simulink model "InnerOuter_Sim_newNav"  (Simulink 7.8)
settings: Solver=ode4  StartTime=0.0  StopTime=300  FixedStep=SampleT  RelTol=1e-3
InitFcn:
  | clc
  | innerOuterInit
values from neighbouring files (symbols this model uses):
  apSampleTime = 0.01    [innerOuterInit.m]
  SampleT = 0.005    [innerOuterInit.m]
  T = 0.01    [innerOuterInit.m]
undefined symbols (not defined in the file or in its folder): A1, Apolar, baseHeight, BasePoint, baseTemp, CD0, chord, CL0, CLa, CLa_dot, Clb, ClDa, CLDe, CLDf, ClDr, clock, Clp, CLq, Clr, Cm0, Cma, CmDe, CmDf, Cmq, Cnb, CnDa, CnDr, Cnp, Cnr, compensatorOn, CYb, CYDr, da_failamp, da_failbias, da_failper, daL_fail, daR_fail, deg, DiscIntNeverNeededParam, dr_fail, dr_failamp, dr_failbias, dr_failper, Earth, elarm, Euler_0, F, gaind, Init_onlyOnce, Init_Reset, ISA_g, Ixx, Iyy, Izz, L1OF, lapseRate, Light, mass, MIL, MinThK ... (+21)
libraries: simulink x69, aerolibconvert2 x19, SLUGS_Library x10, aerolibactuator x5, aerolibobsolete x3, dspmtrx3 x3, aerolibwind2 x2, aerolibtransform2 x1, aerolibatmos2 x1, dsPICdrivers x1
(part 2 of 3)

== system InnerOuter_Sim_newNav/BaroTest/Compute Barometric Height ==
  Base Height (m) : Inport
  Base Pressure (Pa) : Inport  Port=2
  Baro (Pa) : Inport  Port=3
  Constant2 : Constant  Value=baseTemp/(-LapseRate)  OutDataTypeStr=single
  Constant3 : Constant  Value=9.350253e-2  OutDataTypeStr=single
  Constant4 : Constant  Value=-1.888933e-1  OutDataTypeStr=single
  Constant5 : Constant  Value=2.180313e-5  OutDataTypeStr=single
  Divide : Product  Inputs=*/  OutDataTypeStr=single
  Divide{1..4} (4 alike) : Product  OutDataTypeStr=single
  Length Conversion : aerolibconvert2/Length Conversion  IU=ft  OU=m
  Sum1 : Sum  Inputs=|++  OutDataTypeStr=single
  Sum2 : Sum  Inputs=|+-  OutDataTypeStr=single
  Sum3 : Sum  Inputs=3  OutDataTypeStr=single
  "Altitude, m" : Outport
  wires:
  Length Conversion/1 -> Sum1/1
  Sum2/1 -> Divide/1
  Sum1/1 -> "Altitude, m"/1
  Divide3/1 -> Length Conversion/1
  Constant2/1 -> Divide3/2
  Sum3/1 -> Divide3/1
  Constant5/1 -> Sum3/3
  Divide2/1 -> Sum3/2
  Divide1/1 -> Sum3/1
  Constant4/1 -> Divide2/2
  Constant3/1 -> Divide1/2
  Divide4/1 -> Divide1/1  "x^2"
  Divide/1 -> Divide2/1, Divide4/1, Divide4/2  "x"
  Base Pressure (Pa)/1 -> Divide/2, Sum2/2
  Base Height (m)/1 -> Sum1/2
  Baro (Pa)/1 -> Sum2/1

== system InnerOuter_Sim_newNav/BaroTest/Initial Baro Bias ==
  Baro (Pa) : Inport
  Enable : EnablePort
  Data Type Conversion : DataTypeConversion  OutDataTypeStr=double
  Data Type Conversion1 : DataTypeConversion  OutDataTypeStr=single
  Low Pass8 : Subsystem  mask(DiscretizedZeroPole){Zeros=[], Poles=[-3], Gain=3, AbsTol=auto, SampleTime=.01, method=tustin, Wc=1}
      mask prompts: Zeros "Zeros (enter in s-main:)"; Poles "Poles (enter in s-domain:)"; Gain "Gain (enter in s-domain:)"; AbsTol "Absolute tolerance:"; SampleTime "Sample time:"; Wc "Critical Frequency (Hz):"
      mask help: Continuous mask uses c2d to transform parameters onto the Discrete Zero-Pole block inside.
      mask init:
      | st=SampleTime;
      | if length(st)>1
      |     st=SampleTime(1);
      | end
      | if(st>0)
      |     [zerosd,polesd,gaind] = sldiscutil('disczpk', {st,method,Wc,Zeros,Poles,Gain});
      | end	
      | s = get_param(gcb,'maskvalues');
      | zeross = s{1};
      | poless = s{2};
      | gainss = s{3};
      | %zerosc = eval(zeross);
      | %polesc = eval(poless);
      | %gainsc = eval(gainss);
      | sldiscutil('initzpkmask', st);
      | if(st==0)
      | set_param([gcb '/Zero Pole'], 'AbsoluteTolerance', AbsTol);
      | end
      mask StyleString: edit,edit,edit,edit,edit,popup(zoh|foh|tustin|prewarp|matched),edit
      mask CallbackString: |||||hidecrit|
      mask Display:
      | droots(zeross,poless,gainss)
      | text( 0.5, 1.0, method, 'verticalAlignment','top')
  Mux : Mux  Inputs=2
  Scope : Scope
      settings: SaveName=ScopeData8
  "[80k - 120k]" : Saturate  UpperLimit=120000  LowerLimit=80000
  Baro (Gnd) : Outport
  wires:
  Baro (Pa)/1 -> Data Type Conversion/1
  Low Pass8/1(Out1) -> Data Type Conversion1/1
  Data Type Conversion/1 -> Low Pass8/1(In1)
  Data Type Conversion1/1 -> Mux/2, "[80k - 120k]"/1
  Mux/1 -> Scope/1
  "[80k - 120k]"/1 -> Baro (Gnd)/1, Mux/1

== system InnerOuter_Sim_newNav/BaroTest/Zero Out Height ==
  Base Height : Inport
  Computed Height : Inport  Port=2
  Enable : EnablePort
  Integer Delay : Delay  DelayLength=1  InitialCondition=0  InputProcessing=Inherited  SampleTime=.01
  Sum : Sum  Inputs=|+-  OutDataTypeStr=single
  Height Offset : Outport
  wires:
  Computed Height/1 -> Integer Delay/1
  Sum/1 -> Height Offset/1
  Integer Delay/1 -> Sum/2
  Base Height/1 -> Sum/1

== system InnerOuter_Sim_newNav/Create ISR Location From WPs/get sim WP Coord from Index ==
  WP Idx : Inport
  Data Type Conversion : DataTypeConversion  OutDataTypeStr=double
  Data Type Conversion1 : DataTypeConversion  OutDataTypeStr=single
  MATLAB Fcn : MATLABFcn  MATLABFcn=Xpoints(u(1))  OutputDimensions=1  OutputSignalType=real
  MATLAB Fcn1 : MATLABFcn  MATLABFcn=Ypoints(u(1))  OutputDimensions=1
  MATLAB Fcn2 : MATLABFcn  MATLABFcn=Zpoints(u(1))  OutputDimensions=1
  Mux : Mux  Inputs=3
  WP Coord : Outport
  wires:
  Data Type Conversion/1 -> MATLAB Fcn2/1, MATLAB Fcn/1, MATLAB Fcn1/1
  MATLAB Fcn/1 -> Mux/1
  MATLAB Fcn1/1 -> Mux/2
  MATLAB Fcn2/1 -> Mux/3
  WP Idx/1 -> Data Type Conversion/1
  Mux/1 -> Data Type Conversion1/1
  Data Type Conversion1/1 -> WP Coord/1

== system InnerOuter_Sim_newNav/L1 Output Feedback Controller With  Projection Operator/Control  Law ==
  a : Inport
  u : Inport  Port=2
  Compute Coef : Subsystem
  Detect Change : Subsystem
  Divide : Product  SampleTime=apSampleTime
  Divide1 : Product  SampleTime=apSampleTime
  IC : InitialCondition
  Integer Delay : Delay  DelayLength=1  InputProcessing=Inherited  SampleTime=apSampleTime
  Integer Delay1 : Delay  DelayLength=1  InputProcessing=Inherited  SampleTime=apSampleTime
  Subtract : Sum  SampleTime=apSampleTime
  y : Outport
  wires:
  Integer Delay1/1 -> Divide1/2
  u/1 -> Integer Delay/1
  IC/1 -> Compute Coef/Enable
  Subtract/1 -> Integer Delay1/1, y/1
  Divide1/1 -> Subtract/2
  Divide/1 -> Subtract/1
  Integer Delay/1 -> Divide/2
  Detect Change/1(change?) -> IC/1
  Compute Coef/2(c) -> Divide1/1
  Compute Coef/1(b) -> Divide/1
  a/1 -> Detect Change/1(Data), Compute Coef/1(a)

== system InnerOuter_Sim_newNav/L1 Output Feedback Controller With  Projection Operator/Projection Operator ==
  Theta Max : Inport
  Eps 0 : Inport  Port=2
  Theta : Inport  Port=3
  y : Inport  Port=4
  Compare To Zero : simulink/Logic and Bit Operations/Compare To Zero  relop=>=  OutDataTypeStr=boolean  ZeroCross=off
  Compare To Zero1 : simulink/Logic and Bit Operations/Compare To Zero  relop=>  OutDataTypeStr=boolean  ZeroCross=off
  Data Type Conversion1 : DataTypeConversion
  Divide2 : Product  OutDataTypeStr=single
  Enabled Subsystem : Subsystem  TreatAsAtomicUnit=on
  Enabled Subsystem1 : Subsystem  TreatAsAtomicUnit=on
  Enabled Subsystem2 : Subsystem  TreatAsAtomicUnit=on
  F(theta) : Subsystem
  Logical Operator : Logic  Operator=NOT  AllPortsSameDT=off  OutDataTypeStr=uint(8)
  Logical Operator2 : Logic  AllPortsSameDT=off  OutDataTypeStr=uint(8)
  Merge : Merge  InitialOutput=0
  Scope1 : Scope  NumInputPorts=4
      settings: YMin=-0.6~-0.5~-100~-10  YMax=0~5~10~10  SaveName=ScopeData4
  Scope2 : Scope  NumInputPorts=2
      settings: TimeRange=400  YMin=-0.06~-0.06  YMax=0.06~0.06  SaveName=ScopeData15
  "y " : InportShadow  Port=4
  "y    " : InportShadow  Port=4
  "Proj(the, y)" : Outport
  wires:
  Enabled Subsystem1/1(Out1) -> Merge/2
  "y    "/1 -> Enabled Subsystem1/1(y), Enabled Subsystem2/1(y), Scope1/2
  Logical Operator/1 -> Enabled Subsystem/Enable, Scope2/2
  Logical Operator2/1 -> Logical Operator/1, Enabled Subsystem1/Enable, Enabled Subsystem2/Enable, Scope2/1
  Compare To Zero1/1 -> Logical Operator2/1
  F(theta)/2(dif_f_theta) -> Divide2/1, Enabled Subsystem1/3(grad), Enabled Subsystem2/3(grad), Scope1/4
  Compare To Zero/1 -> Logical Operator2/2
  Enabled Subsystem/1(Out1) -> Data Type Conversion1/1
  "y "/1 -> Enabled Subsystem/1(In1)
  Merge/1 -> "Proj(the, y)"/1
  Divide2/1 -> Compare To Zero1/1
  y/1 -> Divide2/2
  F(theta)/1(f_theta) -> Compare To Zero/1, Enabled Subsystem1/2(f_the), Enabled Subsystem2/2(f_the), Scope1/3
  Theta/1 -> F(theta)/3(Theta)
  Eps 0/1 -> F(theta)/2(Eps 0)
  Theta Max/1 -> F(theta)/1(Theta Max)
  Data Type Conversion1/1 -> Merge/1
  Enabled Subsystem2/1(Out1) -> Scope1/1

== system InnerOuter_Sim_newNav/L1 Output Feedback Controller With  Projection Operator/State Predictor ==
  a : Inport
  u : Inport  Port=2
  Compute Coef : Subsystem
  Detect Change : Subsystem
  Divide : Product  SampleTime=apSampleTime
  Divide1 : Product  SampleTime=apSampleTime
  IC : InitialCondition
  Integer Delay : Delay  DelayLength=1  InputProcessing=Inherited  SampleTime=apSampleTime
  Integer Delay1 : Delay  DelayLength=1  InputProcessing=Inherited  SampleTime=apSampleTime
  Subtract : Sum  SampleTime=apSampleTime
  y : Outport
  wires:
  a/1 -> Compute Coef/1(a), Detect Change/1(Data)
  Compute Coef/1(b) -> Divide/1
  Compute Coef/2(c) -> Divide1/1
  Detect Change/1(change?) -> IC/1
  Integer Delay/1 -> Divide/2
  Divide/1 -> Subtract/1
  Divide1/1 -> Subtract/2
  Subtract/1 -> y/1, Integer Delay1/1
  IC/1 -> Compute Coef/Enable
  u/1 -> Integer Delay/1
  Integer Delay1/1 -> Divide1/2

== system InnerOuter_Sim_newNav/L1 Output Feedback Controller With  Projection Operator/Trapezoidal Integrator ==
  x : Inport
  Reset : Inport  Port=2
  Constant : Constant  Value=1/3  OutDataTypeStr=single
  Constant1 : Constant  Value=4/3  OutDataTypeStr=single
  Constant2 : Constant  Value=T/2  OutDataTypeStr=single
  Constant3 : Constant  Value=1/3  OutDataTypeStr=single
  Constant5 : Constant  Value=0  OutDataTypeStr=single
  Integer Delay : Delay  DelayLength=1  InputProcessing=Inherited  SampleTime=T
  Integer Delay1 : Delay  InputProcessing=Inherited  SampleTime=T
  Integer Delay2 : Delay  DelayLength=1  InputProcessing=Inherited  SampleTime=T
  Product{,1..3} (4 alike) : Product  OutDataTypeStr=single  RndMeth=Zero
  Protect NaNs : Subsystem
  Protect NaNs1 : Subsystem
  Subtract : Sum  Inputs=3  OutDataTypeStr=single
  Subtract1 : Sum  Inputs=2  OutDataTypeStr=single
  Switch1 : Switch  Criteria=u2 > Threshold  Threshold=0.3  SampleTime=.01
  "[min max]" : Saturate  UpperLimit=upperLimit  LowerLimit=lowerLimit  SampleTime=T
  Int(x) : Outport
  wires:
  Protect NaNs1/1(Out1) -> Integer Delay2/1, Int(x)/1
  Protect NaNs/1(Out1) -> Integer Delay1/1, Integer Delay/1, Product/1
  Subtract1/1 -> "[min max]"/1
  Product3/1 -> Subtract1/2
  "[min max]"/1 -> Switch1/3
  Switch1/1 -> Protect NaNs1/1(In1)
  Reset/1 -> Switch1/2
  Constant5/1 -> Switch1/1
  Integer Delay2/1 -> Subtract1/1
  Subtract/1 -> Product3/2
  Constant2/1 -> Product3/1
  Product2/1 -> Subtract/3
  Product1/1 -> Subtract/2
  Product/1 -> Subtract/1
  x/1 -> Protect NaNs/1(In1)
  Constant3/1 -> Product2/2
  Integer Delay1/1 -> Product2/1
  Integer Delay/1 -> Product1/1
  Constant1/1 -> Product1/2
  Constant/1 -> Product/2

== system InnerOuter_Sim_newNav/PT Unit (Vlad) /LPF the Euler and Construct Matrix ==
  Euler : Inport
  Euler Angles to  Direction Cosine Matrix : aerolibobsolete/Euler Angles to  Direction Cosine Matrix
  Terminator : Terminator
  "Tustin Lowpass, Auto Initial Condition1" : Subsystem  mask(Tustin1stOrderLowpassAutoInitialCondition){f=75, T=T}
      mask prompts: f "Lowpass Frequency"; T "Sample Time"
      mask help: Takes a 3db rolloff frequency (in Hz, NOT radians/s) and a sample time. Performs a symbolic Tustin conversion and implements in a discrete filter. The initial output of the filter is set by the first sample.
      mask Help: Enter the desired 3db rolloff frequency in Hz and the sample time. Initial conditions are sampled automatically.
      mask Display: fprintf('%.2f Hz lowpass',f)
  "Tustin Lowpass, Auto Initial Condition2" : Subsystem  mask(Tustin1stOrderLowpassAutoInitialCondition){f=75, T=T}
      mask prompts: f "Lowpass Frequency"; T "Sample Time"
      mask help: Takes a 3db rolloff frequency (in Hz, NOT radians/s) and a sample time. Performs a symbolic Tustin conversion and implements in a discrete filter. The initial output of the filter is set by the first sample.
      mask Help: Enter the desired 3db rolloff frequency in Hz and the sample time. Initial conditions are sampled automatically.
      mask Display: fprintf('%.2f Hz lowpass',f)
  "Tustin Lowpass, Auto Initial Condition3" : Subsystem  mask(Tustin1stOrderLowpassAutoInitialCondition){f=75, T=T}
      mask prompts: f "Lowpass Frequency"; T "Sample Time"
      mask help: Takes a 3db rolloff frequency (in Hz, NOT radians/s) and a sample time. Performs a symbolic Tustin conversion and implements in a discrete filter. The initial output of the filter is set by the first sample.
      mask Help: Enter the desired 3db rolloff frequency in Hz and the sample time. Initial conditions are sampled automatically.
      mask Display: fprintf('%.2f Hz lowpass',f)
  "[a b c]" : Demux  Outputs=3
  myMux Fun5 : MATLAB Function  TreatAsAtomicUnit=on
  Rfg2b : Outport
  wires:
  myMux Fun5/1(y) -> Terminator/1
  Euler/1 -> Euler Angles to  Direction Cosine Matrix/1, "[a b c]"/1
  "[a b c]"/3 -> "Tustin Lowpass, Auto Initial Condition3"/1(In1)
  "[a b c]"/2 -> "Tustin Lowpass, Auto Initial Condition1"/1(In1)
  "[a b c]"/1 -> "Tustin Lowpass, Auto Initial Condition2"/1(In1)
  "Tustin Lowpass, Auto Initial Condition3"/1(Out1) -> myMux Fun5/3(u3)
  "Tustin Lowpass, Auto Initial Condition1"/1(Out1) -> myMux Fun5/2(u2)
  "Tustin Lowpass, Auto Initial Condition2"/1(Out1) -> myMux Fun5/1(u1)
  Euler Angles to  Direction Cosine Matrix/1 -> Rfg2b/1

== system InnerOuter_Sim_newNav/Simple Car Model/Heading/Speed to Velocity ==
  Heading : Inport
  Speed : Inport  Port=2
  Add : Sum  Inputs=+-
  Angle Conversion : aerolibconvert2/Angle Conversion  IU=deg  OU=rad
  Divide : Product
  Divide1 : Product
  Low pass the  change of direction : Subsystem  mask(Tustin1stOrderLowpassAutoInitialCondition){f=0.05, T=apSampleTime}
      mask prompts: f "Lowpass Frequency"; T "Sample Time"
      mask help: Takes a 3db rolloff frequency (in Hz, NOT radians/s) and a sample time. Performs a symbolic Tustin conversion and implements in a discrete filter. The initial output of the filter is set by the first sample.
      mask Help: Enter the desired 3db rolloff frequency in Hz and the sample time. Initial conditions are sampled automatically.
      mask Display: fprintf('%.2f Hz lowpass',f)
  Mux : Mux  Inputs=3
  Rate Transition1 : RateTransition  OutPortSampleTime=apSampleTime
  Rate Transition2 : RateTransition  OutPortSampleTime=apSampleTime
  Speed1 : Constant  Value=0
  Speed2 : Constant  Value=450*pi/180  SampleTime=0.01
  Trigonometric Function : Trigonometry  Operator=cos
  Trigonometric Function1 : Trigonometry
  Velocity : Outport
  wires:
  Speed1/1 -> Mux/3
  Speed2/1 -> Add/1
  Add/1 -> Trigonometric Function/1, Trigonometric Function1/1  "alpha"
  Trigonometric Function/1 -> Divide/1
  Speed/1 -> Rate Transition2/1
  Divide/1 -> Mux/1
  Angle Conversion/1 -> Add/2
  Divide1/1 -> Mux/2
  Trigonometric Function1/1 -> Divide1/2
  Low pass the  change of direction/1(Out1) -> Angle Conversion/1
  Heading/1 -> Rate Transition1/1
  Mux/1 -> Velocity/1
  Rate Transition1/1 -> Low pass the  change of direction/1(In1)
  Rate Transition2/1 -> Divide1/1, Divide/2

== system InnerOuter_Sim_newNav/Simple Car Model/Simple Car Model ==
  Velocity : Inport
  Constant13 : Constant  Value=BasePoint  OutDataTypeStr=single
  Data Type Conversion : DataTypeConversion  OutDataTypeStr=single
  Data Type Conversion1 : DataTypeConversion  OutDataTypeStr=single
  Discrete-Time Integrator : DiscreteIntegrator  InitialConditionSource=external  SampleTime=0.01  ICPrevOutput=DiscIntNeverNeededParam  ICPrevScaledInput=DiscIntNeverNeededParam
  p_cg : Outport
  wires:
  Velocity/1 -> Data Type Conversion1/1
  Constant13/1 -> Discrete-Time Integrator/2
  Discrete-Time Integrator/1 -> Data Type Conversion/1
  Data Type Conversion/1 -> p_cg/1
  Data Type Conversion1/1 -> Discrete-Time Integrator/1

== system InnerOuter_Sim_newNav/6DOF Model/Plant/6-DOF EOM ==
  "[F,M]" : Inport
  Vb Corr : Inport  Port=2
  Angular Rates : Integrator  InitialCondition=PQR_0'
  Demux1 : Demux  Outputs=2
  Euler Angles : Integrator  InitialCondition=Euler_0
  Get Euler Dot : Subsystem
      mask Display:
      | port_label('input', 1, 'p, q, r')
      | port_label('input', 2, 'Euler')
      | port_label('output', 1, 'Euler_dot')
  Mux : Mux  Inputs=[3;3]
  NED2NEU : Gain  Gain=[1 0 0;0 1 0;0 0 -1]  Multiplication=Matrix(K*u)  SaturateOnIntegerOverflow=on  OutDataTypeStr=Inherit: Same as input  ParamDataTypeStr=Inherit: Same as input
  Position : Integrator  InitialCondition=Pos_0'
  RB2L * Vb : Product  Multiplication=Matrix(*)  SaturateOnIntegerOverflow=on  InputSameDT=on  OutDataTypeStr=Inherit: Same as first input
  RB2LTP : Subsystem
  Velocities Body : Integrator  InitialCondition=Vb_0'
  "[V1,2,3,W1,2,3]" : Subsystem
  X,Y,Z (LTP) : Outport
  "Vx, Vy, Vz" : Outport  Port=2
  Euler : Outport  Port=3
  "p, q, r" : Outport  Port=4
  Vb : Outport  Port=5
  Ab meas : Outport  Port=6
  Euler_dot : Outport  Port=7
  wires:
  "[V1,2,3,W1,2,3]"/1("Acc_meas ") -> Ab meas/1
  Euler Angles/1 -> "[V1,2,3,W1,2,3]"/2(Euler), Get Euler Dot/2(Euler), Euler/1, RB2LTP/1(Euler)
  Demux1/1 -> Velocities Body/1
  "[V1,2,3,W1,2,3]"/2(V*dot) -> Demux1/1
  Demux1/2 -> Angular Rates/1
  "[F,M]"/1 -> "[V1,2,3,W1,2,3]"/1("[F ; M]")
  RB2LTP/1(Rot) -> RB2L * Vb/1
  Velocities Body/1 -> Vb/1, RB2L * Vb/2
  Mux/1 -> "[V1,2,3,W1,2,3]"/3(V*)
  Position/1 -> X,Y,Z (LTP)/1
  Angular Rates/1 -> Get Euler Dot/1(p,q,r), Mux/2, "p, q, r"/1
  RB2L * Vb/1 -> NED2NEU/1, "Vx, Vy, Vz"/1  "NED"
  NED2NEU/1 -> Position/1
  Get Euler Dot/1(Euler_dot) -> Euler Angles/1, Euler_dot/1
  Vb Corr/1 -> Mux/1

== system InnerOuter_Sim_newNav/6DOF Model/Plant/Engine Model ==
  dt : Inport
  Vmag : Inport  Port=2
  Constant4 : Constant  Value=0
  Get To1 : Subsystem
  Mux : Mux  Inputs=2
  Mux1 : Mux  Inputs=3
  Thrust Available (lbs) : Fcn  Expr=u(1) - 0.047*sqrt(u(1))*u(2)
  kg2N : Gain  Gain=ISA_g  SaturateOnIntegerOverflow=on  OutDataTypeStr=Inherit: Same as input  ParamDataTypeStr=Inherit: Same as input
  lbs2kg : Gain  Gain=0.45359237  SaturateOnIntegerOverflow=on  OutDataTypeStr=Inherit: Same as input  ParamDataTypeStr=Inherit: Same as input
  Thrust : Outport
  wires:
  dt/1 -> Get To1/1(dt)
  Get To1/1(To) -> Mux/1
  Mux/1 -> Thrust Available (lbs)/1
  Thrust Available (lbs)/1 -> lbs2kg/1
  Vmag/1 -> Mux/2
  Mux1/1 -> Thrust/1
  lbs2kg/1 -> kg2N/1
  Constant4/1 -> Mux1/2, Mux1/3
  kg2N/1 -> Mux1/1

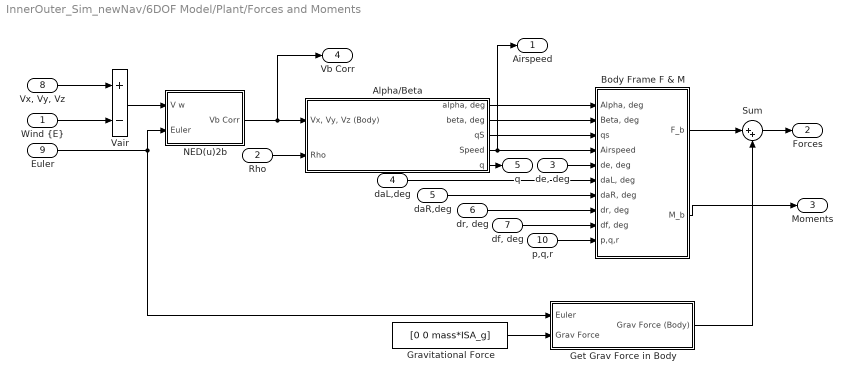
== system InnerOuter_Sim_newNav/6DOF Model/Plant/Forces and Moments ==
  "Wind {E}" : Inport
  Rho : Inport  Port=2
  "de, deg" : Inport  Port=3
  daL,deg : Inport  Port=4
  daR,deg : Inport  Port=5
  "dr, deg" : Inport  Port=6
  "df, deg" : Inport  Port=7
  "Vx, Vy, Vz " : Inport  Port=8
  Euler : Inport  Port=9  PortDimensions=3
  p,q,r : Inport  Port=10
  Alpha/Beta : Subsystem
  Body Frame F & M : Subsystem
  Get Grav Force in Body : Subsystem
  Gravitational Force : Constant  Value=[0 0 mass*ISA_g]  VectorParams1D=off
  NED(u)2b : Subsystem
  Sum : Sum  Inputs=|++  SaturateOnIntegerOverflow=on
  Vair : Sum  Inputs=+-  SaturateOnIntegerOverflow=on  InputSameDT=on  OutDataTypeStr=Inherit: Same as first input
  Airspeed : Outport
  Forces : Outport  Port=2
  Moments : Outport  Port=3
  Vb Corr : Outport  Port=4
  q : Outport  Port=5
  wires:
  Get Grav Force in Body/1(Grav Force (Body)) -> Sum/2
  Alpha/Beta/5(q) -> q/1
  "Vx, Vy, Vz "/1 -> Vair/1
  Vair/1 -> NED(u)2b/1(V w)
  Euler/1 -> NED(u)2b/2(Euler), Get Grav Force in Body/1(Euler)
  Rho/1 -> Alpha/Beta/2(Rho)
  NED(u)2b/1(Vb Corr) -> Alpha/Beta/1("Vx, Vy, Vz (Body)"), Vb Corr/1
  Body Frame F & M/2(M_b) -> Moments/1
  Gravitational Force/1 -> Get Grav Force in Body/2(Grav Force)
  Body Frame F & M/1(F_b) -> Sum/1
  Sum/1 -> Forces/1
  Alpha/Beta/3(qS) -> Body Frame F & M/3(qs)
  Alpha/Beta/4(Speed) -> Body Frame F & M/4(Airspeed), Airspeed/1
  "df, deg"/1 -> Body Frame F & M/9("df, deg")
  p,q,r/1 -> Body Frame F & M/10(p,q,r)
  Alpha/Beta/2("beta, deg") -> Body Frame F & M/2("Beta, deg")
  "dr, deg"/1 -> Body Frame F & M/8("dr, deg")
  daL,deg/1 -> Body Frame F & M/6("daL, deg")
  Alpha/Beta/1("alpha, deg") -> Body Frame F & M/1("Alpha, deg")
  "de, deg"/1 -> Body Frame F & M/5("de, deg")
  "Wind {E}"/1 -> Vair/2
  daR,deg/1 -> Body Frame F & M/7("daR, deg")

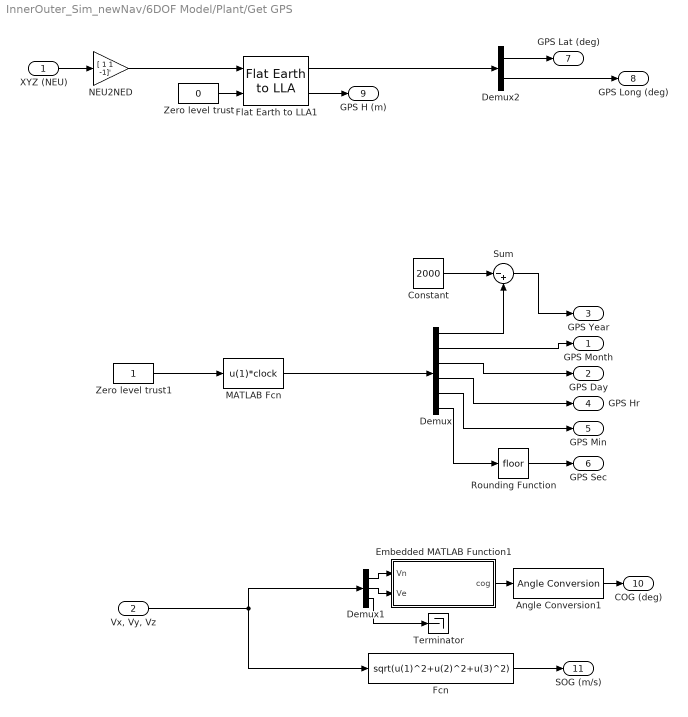
== system InnerOuter_Sim_newNav/6DOF Model/Plant/Get GPS ==
  XYZ (NEU) : Inport
  "Vx, Vy, Vz" : Inport  Port=2
  Angle Conversion1 : aerolibconvert2/Angle Conversion  IU=rad  OU=deg
  Constant : Constant  Value=2000
  Demux : Demux  Outputs=6
  Demux1 : Demux  Outputs=3
  Demux2 : Demux  Outputs=2
  Embedded MATLAB Function1 : MATLAB Function  TreatAsAtomicUnit=on
  Fcn : Fcn  Expr=sqrt(u(1)^2+u(2)^2+u(3)^2)
  Flat Earth to LLA1 : aerolibtransform2/Flat Earth to LLA  units=Metric (MKS)  ptype=Earth (WGS84)  F=1/298.257223563  R=6378137  LL0=[0 10]  psi=0
  MATLAB Fcn : MATLABFcn  MATLABFcn=u(1)*clock  OutputSignalType=real  SampleTime=SampleT
  NEU2NED : Gain  Gain=[ 1 1 -1]'  SaturateOnIntegerOverflow=on  OutDataTypeStr=Inherit: Same as input  ParamDataTypeStr=Inherit: Same as input
  Rounding Function : Rounding
  Sum : Sum  Inputs=|-+
  Terminator : Terminator
  Zero level trust : Constant  Value=0  SampleTime=SampleT
  Zero level trust1 : Constant  SampleTime=SampleT
  GPS Month : Outport
  GPS Day : Outport  Port=2
  GPS Year : Outport  Port=3
  GPS Hr : Outport  Port=4
  GPS Min : Outport  Port=5
  GPS Sec : Outport  Port=6
  GPS Lat (deg) : Outport  Port=7
  GPS Long (deg) : Outport  Port=8
  GPS H (m) : Outport  Port=9
  COG (deg) : Outport  Port=10
  SOG (m/s) : Outport  Port=11
  wires:
  NEU2NED/1 -> Flat Earth to LLA1/1
  Zero level trust/1 -> Flat Earth to LLA1/2
  XYZ (NEU)/1 -> NEU2NED/1
  Flat Earth to LLA1/1 -> Demux2/1
  Flat Earth to LLA1/2 -> GPS H (m)/1
  Zero level trust1/1 -> MATLAB Fcn/1
  MATLAB Fcn/1 -> Demux/1
  Demux/2 -> GPS Month/1
  Demux/3 -> GPS Day/1
  Demux/4 -> GPS Hr/1
  Demux/5 -> GPS Min/1
  Demux/6 -> Rounding Function/1
  Rounding Function/1 -> GPS Sec/1
  Demux2/1 -> GPS Lat (deg)/1
  Demux2/2 -> GPS Long (deg)/1
  Fcn/1 -> SOG (m/s)/1
  Demux1/1 -> Embedded MATLAB Function1/1(Vn)
  Demux1/2 -> Embedded MATLAB Function1/2(Ve)
  "Vx, Vy, Vz"/1 -> Demux1/1, Fcn/1
  Embedded MATLAB Function1/1(cog) -> Angle Conversion1/1
  Angle Conversion1/1 -> COG (deg)/1
  Demux/1 -> Sum/2
  Constant/1 -> Sum/1
  Sum/1 -> GPS Year/1
  Demux1/3 -> Terminator/1

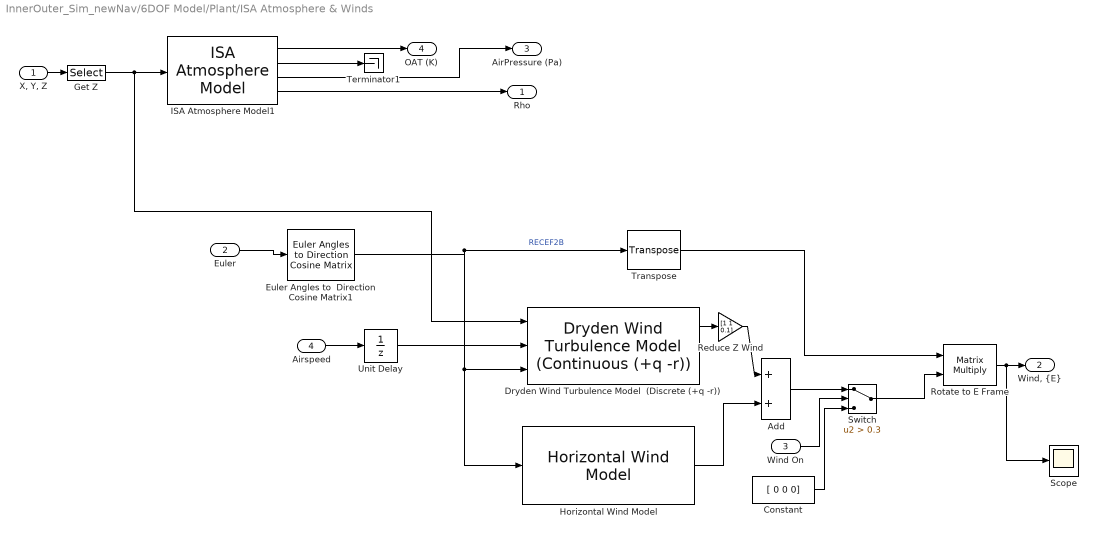
== system InnerOuter_Sim_newNav/6DOF Model/Plant/ISA Atmosphere & Winds ==
  "X, Y, Z" : Inport
  Euler : Inport  Port=2
  Wind On : Inport  Port=3
  Airspeed : Inport  Port=4
  Add : Sum  Inputs=2
  Constant : Constant  Value=[ 0 0 0]
  Dryden Wind Turbulence Model  (Discrete (+q -r)) : aerolibwind2/Dryden Wind Turbulence Model  (Continuous (+q -r))  units=Metric (MKS)  spec=MIL-F-8785C  model=Discrete Dryden (+q -r)  W20=windBase*0.3  Wdeg=windDirTurb  TurbProb=10^-2 - Light  L_high=533.4  Wingspan=span  ts=0.005  Seed=[23341 23342 23343 23344]  T_on=on
  Euler Angles to  Direction Cosine Matrix1 : aerolibobsolete/Euler Angles to  Direction Cosine Matrix
  Get Z : Selector  InputPortWidth=3  IndexOptions=Index vector (dialog)  Indices=[3]  OutputSizes=[(-2)]
  Horizontal Wind Model : aerolibwind2/Horizontal Wind Model  units=Metric (MKS)  Vw_source=Internal  Vwind=windBase  W_source=Internal  Wdeg=windDirHor
  ISA Atmosphere Model1 : aerolibatmos2/ISA Atmosphere Model  custom=off  g=9.80665  gamma=1.4  R=287.0531  L=0.0065  h_trop=11000  h_strat=20000  rho0=1.225  P0=101325  T0=288.15
  Reduce Z Wind : Gain  Gain=[1 1 0.1]
  Rotate to E Frame : Product  Multiplication=Matrix(*)
  Scope : Scope
      settings: YMin=-1  YMax=13  SaveName=windData  DataFormat=Array
  Switch : Switch  Criteria=u2 > Threshold  Threshold=0.3
  Terminator1 : Terminator
  Transpose : dspmtrx3/Transpose  Hermitian=off  overflowFlag=off
  Unit Delay : UnitDelay  SampleTime=-1
  Rho : Outport
  "Wind, {E}" : Outport  Port=2
  AirPressure (Pa) : Outport  Port=3
  OAT (K) : Outport  Port=4
  wires:
  "X, Y, Z"/1 -> Get Z/1
  Get Z/1 -> ISA Atmosphere Model1/1, Dryden Wind Turbulence Model  (Discrete (+q -r))/1
  ISA Atmosphere Model1/4 -> Rho/1
  ISA Atmosphere Model1/1 -> OAT (K)/1
  ISA Atmosphere Model1/2 -> Terminator1/1
  ISA Atmosphere Model1/3 -> AirPressure (Pa)/1
  Euler/1 -> Euler Angles to  Direction Cosine Matrix1/1
  Euler Angles to  Direction Cosine Matrix1/1 -> Dryden Wind Turbulence Model  (Discrete (+q -r))/3, Horizontal Wind Model/1, Transpose/1  "RECEF2B"
  Airspeed/1 -> Unit Delay/1
  Add/1 -> Switch/1
  Unit Delay/1 -> Dryden Wind Turbulence Model  (Discrete (+q -r))/2
  Horizontal Wind Model/1 -> Add/2
  Switch/1 -> Rotate to E Frame/2
  Wind On/1 -> Switch/2
  Constant/1 -> Switch/3
  Transpose/1 -> Rotate to E Frame/1
  Rotate to E Frame/1 -> "Wind, {E}"/1, Scope/1
  Dryden Wind Turbulence Model  (Discrete (+q -r))/1 -> Reduce Z Wind/1
  Reduce Z Wind/1 -> Add/1

== system InnerOuter_Sim_newNav/6DOF Model/Plant/Magnetometer ==
  Euler : Inport
  LTP2B : dspmtrx3/Transpose  Hermitian=off  overflowFlag=off
  Mag Field in nT source:  http://www.ngdc.noaa.gov/geomagmodels/struts/calcIGRFWMM : Constant  Value=magField
  Product : Product  Multiplication=Matrix(*)  RndMeth=Zero
  RB2LTP : Subsystem
  "Mag, nT" : Outport
  wires:
  RB2LTP/1(Rot) -> LTP2B/1
  LTP2B/1 -> Product/1
  Mag Field in nT source:  http://www.ngdc.noaa.gov/geomagmodels/struts/calcIGRFWMM/1 -> Product/2
  Euler/1 -> RB2LTP/1(Euler)
  Product/1 -> "Mag, nT"/1

== system InnerOuter_Sim_newNav/6DOF Model/Plant/[0, pi] Wrap Around ==
  Euler : Inport
  Compare To Zero : simulink/Logic and Bit Operations/Compare To Zero  relop=>=  OutDataTypeStr=uint8  ZeroCross=off
  Logical Operator : Logic  Operator=NOT  AllPortsSameDT=off  OutDataTypeStr=boolean
  Merge : Merge
  Mux2 : Mux  Inputs=2
  Negative Yaw : Subsystem
  Positive Yaw : Subsystem
  Selector1 : Selector  InputPortWidth=3  IndexOptions=Index vector (dialog)  Indices=[1 2]  OutputSizes=1
  Selector2 : Selector  InputPortWidth=3  IndexOptions=Index vector (dialog)  Indices=[3]  OutputSizes=1
  Euler-Wrapped : Outport
  wires:
  Euler/1 -> Selector2/1, Selector1/1
  Selector1/1 -> Mux2/1
  Mux2/1 -> Euler-Wrapped/1
  Selector2/1 -> Compare To Zero/1, Positive Yaw/1(yaw), Negative Yaw/1(yaw)
  Compare To Zero/1 -> Positive Yaw/Enable, Logical Operator/1
  Logical Operator/1 -> Negative Yaw/Enable
  Merge/1 -> Mux2/2
  Positive Yaw/1(yaw_wr) -> Merge/1
  Negative Yaw/1(yaw_wr) -> Merge/2

== system InnerOuter_Sim_newNav/6DOF Model/Split Ailerons And Introduce Failures/Aileron Flaping Failure ==
  Pulse Generator1 : DiscretePulseGenerator  PulseType=Time based  Amplitude=da_failamp  Period=da_failper  PulseWidth=50
  Vair2 : Sum  Inputs=+++  SaturateOnIntegerOverflow=on  InputSameDT=on  OutDataTypeStr=Inherit: Same as first input
  da_failbias : Constant  Value=da_failbias
  da_failbias1 : Constant  Value=0
  "da, Fail, deg" : Outport
  wires:
  Pulse Generator1/1 -> Vair2/1
  da_failbias/1 -> Vair2/2
  da_failbias1/1 -> Vair2/3
  Vair2/1 -> "da, Fail, deg"/1

== system InnerOuter_Sim_newNav/6DOF Model/Split Ailerons And Introduce Failures/Rudder Failure ==
  Pulse Generator1 : DiscretePulseGenerator  PulseType=Time based  Amplitude=dr_failamp  Period=dr_failper  PulseWidth=50
  Vair2 : Sum  Inputs=+++  SaturateOnIntegerOverflow=on  InputSameDT=on  OutDataTypeStr=Inherit: Same as first input
  da_failbias : Constant  Value=dr_failbias
  da_failbias1 : Constant  Value=0
  "da, Fail, deg" : Outport
  wires:
  Vair2/1 -> "da, Fail, deg"/1
  da_failbias1/1 -> Vair2/3
  da_failbias/1 -> Vair2/2
  Pulse Generator1/1 -> Vair2/1

== system InnerOuter_Sim_newNav/BaroTest/Initial Baro Bias/Low Pass8 ==
  In1 : Inport
  Discrete Zero-Pole : DiscreteZeroPole  Zeros=zerosd  Poles=polesd  Gain=gaind  SampleTime=SampleTime
  Out1 : Outport
  wires:
  In1/1 -> Discrete Zero-Pole/1
  Discrete Zero-Pole/1 -> Out1/1

== system InnerOuter_Sim_newNav/L1 Output Feedback Controller With  Projection Operator/Control  Law/Compute Coef ==
  a : Inport
  Enable : EnablePort
  -T : Gain  Gain=-apSampleTime  SampleTime=apSampleTime
  1-c : Sum  Inputs=-+  OutDataTypeStr=single  SampleTime=apSampleTime
  Constant : Constant
  Subsystem11 : Subsystem  AncestorBlock=SLUGS_Library/Subsystem11
  b : Outport
  c : Outport  Port=2
  wires:
  a/1 -> -T/1
  1-c/1 -> b/1
  Constant/1 -> 1-c/2
  Subsystem11/1(exp(u)) -> c/1, 1-c/1  "c"
  -T/1 -> Subsystem11/1(u)

== system InnerOuter_Sim_newNav/L1 Output Feedback Controller With  Projection Operator/Control  Law/Detect Change ==
  Data : Inport
  Abs1 : Abs  SampleTime=apSampleTime
  Difference1 : simulink/Discrete/Difference  ICPrevInput=0.0  InputProcessing=Inherited  OutMin=[]  OutMax=[]  OutDataType=sfix(16)  OutScaling=2^-10  DoSatur=off
  Saturation1 : Saturate  UpperLimit=1  LowerLimit=0  SampleTime=apSampleTime
  change? : Outport
  wires:
  Saturation1/1 -> change?/1
  Data/1 -> Difference1/1
  Abs1/1 -> Saturation1/1
  Difference1/1 -> Abs1/1

== system InnerOuter_Sim_newNav/L1 Output Feedback Controller With  Projection Operator/Projection Operator/Enabled Subsystem ==
  In1 : Inport
  Enable : EnablePort
  Out1 : Outport
  wires:
  In1/1 -> Out1/1

== system InnerOuter_Sim_newNav/L1 Output Feedback Controller With  Projection Operator/Projection Operator/Enabled Subsystem1 ==
  y : Inport
  f_the : Inport  Port=2
  grad : Inport  Port=3
  Enable : EnablePort
  Constant : Constant  OutDataTypeStr=single
  Divide1 : Product  OutDataTypeStr=single
  Divide2 : Product  OutDataTypeStr=single
  Sign : Signum
  Subtract : Sum  Inputs=+-  OutDataTypeStr=single
  Out1 : Outport
  wires:
  Divide2/1 -> Out1/1
  y/1 -> Divide2/1
  Subtract/1 -> Divide2/2
  f_the/1 -> Divide1/1
  Constant/1 -> Subtract/1
  Sign/1 -> Divide1/2
  grad/1 -> Sign/1
  Divide1/1 -> Subtract/2

== system InnerOuter_Sim_newNav/L1 Output Feedback Controller With  Projection Operator/Projection Operator/Enabled Subsystem2 ==
  y : Inport
  f_the : Inport  Port=2
  grad : Inport  Port=3
  Enable : EnablePort
  Constant : Constant  OutDataTypeStr=single
  Divide1 : Product  OutDataTypeStr=single
  Divide2 : Product  OutDataTypeStr=single
  Sign : Signum
  Subtract : Sum  Inputs=+-  OutDataTypeStr=single
  Out1 : Outport
  wires:
  Divide1/1 -> Subtract/2
  grad/1 -> Sign/1
  Sign/1 -> Divide1/2
  Constant/1 -> Subtract/1
  f_the/1 -> Divide1/1
  Subtract/1 -> Divide2/2
  y/1 -> Divide2/1
  Divide2/1 -> Out1/1

== system InnerOuter_Sim_newNav/L1 Output Feedback Controller With  Projection Operator/Projection Operator/F(theta) ==
  Theta Max : Inport
  Eps 0 : Inport  Port=2
  Theta : Inport  Port=3
  Constant : Constant  Value=2  OutDataTypeStr=single
  Divide : Product  OutDataTypeStr=single
  Divide1 : Product  OutDataTypeStr=single
  Divide2 : Product  OutDataTypeStr=single
  Divide3 : Product  Inputs=*/  OutDataTypeStr=single
  Divide4 : Product  Inputs=/**  OutDataTypeStr=single
  Subtract : Sum  Inputs=+-  OutDataTypeStr=single
  "Theta " : InportShadow  Port=3
  f_theta : Outport
  dif_f_theta : Outport  Port=2
  wires:
  Divide4/1 -> dif_f_theta/1
  "Theta "/1 -> Divide4/2
  Constant/1 -> Divide4/3
  Divide3/1 -> f_theta/1
  Divide2/1 -> Divide4/1, Divide3/2
  Subtract/1 -> Divide3/1
  Eps 0/1 -> Divide2/2
  Divide1/1 -> Divide2/1, Subtract/2
  Divide/1 -> Subtract/1
  Theta Max/1 -> Divide1/1, Divide1/2
  Theta/1 -> Divide/2, Divide/1

== system InnerOuter_Sim_newNav/L1 Output Feedback Controller With  Projection Operator/State Predictor/Compute Coef ==
  a : Inport
  Enable : EnablePort
  -T : Gain  Gain=-apSampleTime  SampleTime=apSampleTime
  1-c : Sum  Inputs=-+  OutDataTypeStr=single
  Constant : Constant
  Subsystem11 : Subsystem  AncestorBlock=SLUGS_Library/Subsystem11
  b : Outport
  c : Outport  Port=2
  wires:
  -T/1 -> Subsystem11/1(u)
  Subsystem11/1(exp(u)) -> 1-c/1, c/1  "c"
  Constant/1 -> 1-c/2
  1-c/1 -> b/1
  a/1 -> -T/1

== system InnerOuter_Sim_newNav/L1 Output Feedback Controller With  Projection Operator/State Predictor/Detect Change ==
  Data : Inport
  Abs1 : Abs  SampleTime=apSampleTime
  Difference1 : simulink/Discrete/Difference  ICPrevInput=0.0  InputProcessing=Inherited  OutMin=[]  OutMax=[]  OutDataType=sfix(16)  OutScaling=2^-10  DoSatur=off
  Saturation1 : Saturate  UpperLimit=1  LowerLimit=0  SampleTime=apSampleTime
  change? : Outport
  wires:
  Difference1/1 -> Abs1/1
  Abs1/1 -> Saturation1/1
  Data/1 -> Difference1/1
  Saturation1/1 -> change?/1

== system InnerOuter_Sim_newNav/L1 Output Feedback Controller With  Projection Operator/Trapezoidal Integrator/Protect NaNs ==
  In1 : Inport
  Integer Delay3 : Delay  DelayLength=1  InputProcessing=Inherited  SampleTime=T
  Relational Operator2 : RelationalOperator  Operator===  OutDataTypeStr=uint(8)
  Switch3 : Switch  Criteria=u2 > Threshold  Threshold=0.3  SampleTime=.01
  Out1 : Outport
  wires:
  Integer Delay3/1 -> Switch3/3
  Switch3/1 -> Out1/1, Integer Delay3/1
  In1/1 -> Relational Operator2/2, Relational Operator2/1, Switch3/1
  Relational Operator2/1 -> Switch3/2

== system InnerOuter_Sim_newNav/L1 Output Feedback Controller With  Projection Operator/Trapezoidal Integrator/Protect NaNs1 ==
  In1 : Inport
  Integer Delay3 : Delay  DelayLength=1  InputProcessing=Inherited  SampleTime=T
  Relational Operator2 : RelationalOperator  Operator===  OutDataTypeStr=uint(8)
  Switch3 : Switch  Criteria=u2 > Threshold  Threshold=0.3  SampleTime=.01
  Out1 : Outport
  wires:
  Relational Operator2/1 -> Switch3/2
  In1/1 -> Switch3/1, Relational Operator2/1, Relational Operator2/2
  Switch3/1 -> Integer Delay3/1, Out1/1
  Integer Delay3/1 -> Switch3/3

== system InnerOuter_Sim_newNav/PT Unit (Vlad) /LPF the Euler and Construct Matrix/Tustin Lowpass, Auto Initial Condition1 ==
  In1 : Inport
  Constant : Constant  Value=T
  Constant1 : Constant  Value=f
  Embedded MATLAB Function : MATLAB Function  TreatAsAtomicUnit=on
  Out1 : Outport
  wires:
  Constant/1 -> Embedded MATLAB Function/2(T)
  Constant1/1 -> Embedded MATLAB Function/3(f)
  Embedded MATLAB Function/1(y) -> Out1/1
  In1/1 -> Embedded MATLAB Function/1(u)

== system InnerOuter_Sim_newNav/PT Unit (Vlad) /LPF the Euler and Construct Matrix/Tustin Lowpass, Auto Initial Condition2 ==
  In1 : Inport
  Constant : Constant  Value=T
  Constant1 : Constant  Value=f
  Embedded MATLAB Function : MATLAB Function  TreatAsAtomicUnit=on
  Out1 : Outport
  wires:
  In1/1 -> Embedded MATLAB Function/1(u)
  Embedded MATLAB Function/1(y) -> Out1/1
  Constant1/1 -> Embedded MATLAB Function/3(f)
  Constant/1 -> Embedded MATLAB Function/2(T)

== system InnerOuter_Sim_newNav/PT Unit (Vlad) /LPF the Euler and Construct Matrix/Tustin Lowpass, Auto Initial Condition3 ==
  In1 : Inport
  Constant : Constant  Value=T
  Constant1 : Constant  Value=f
  Embedded MATLAB Function : MATLAB Function  TreatAsAtomicUnit=on
  Out1 : Outport
  wires:
  In1/1 -> Embedded MATLAB Function/1(u)
  Embedded MATLAB Function/1(y) -> Out1/1
  Constant1/1 -> Embedded MATLAB Function/3(f)
  Constant/1 -> Embedded MATLAB Function/2(T)

== system InnerOuter_Sim_newNav/Simple Car Model/Heading/Speed to Velocity/Low pass the  change of direction ==
  In1 : Inport
  Constant : Constant  Value=T  SampleTime=T
  Constant1 : Constant  Value=f  SampleTime=T
  Embedded MATLAB Function : MATLAB Function  TreatAsAtomicUnit=on
  Out1 : Outport
  wires:
  Constant/1 -> Embedded MATLAB Function/2(T)
  Constant1/1 -> Embedded MATLAB Function/3(f)
  Embedded MATLAB Function/1(y) -> Out1/1
  In1/1 -> Embedded MATLAB Function/1(u)

== system InnerOuter_Sim_newNav/6DOF Model/Plant/6-DOF EOM/Get Euler Dot ==
  p,q,r : Inport
  Euler : Inport  Port=2
  Mux1 : Mux  Inputs=[3 3]
  Mux2 : Mux  Inputs=3
  phidot : Fcn  Expr=u[1]+u[2]*sin(u[4])*tan(u[5])+u[3]*cos(u[4])*tan(u[5])
  psidot : Fcn  Expr=u[2]*sin(u[4])/cos(u[5])+u[3]*cos(u[4])/cos(u[5])
  thetadot : Fcn  Expr=u[2]*cos(u[4])-u[3]*sin(u[4])
  Euler_dot : Outport
  wires:
  Mux2/1 -> Euler_dot/1
  phidot/1 -> Mux2/1
  thetadot/1 -> Mux2/2
  psidot/1 -> Mux2/3
  Mux1/1 -> thetadot/1, phidot/1, psidot/1
  p,q,r/1 -> Mux1/1
  Euler/1 -> Mux1/2

== system InnerOuter_Sim_newNav/6DOF Model/Plant/6-DOF EOM/RB2LTP ==
  Euler : Inport
  11 : Fcn  Expr=cos(u[3])*cos(u[2])
  12 : Fcn  Expr=sin(u[3])*cos(u[2])
  13 : Fcn  Expr=-sin(u[2])
  21 : Fcn  Expr=cos(u[3])*sin(u[2])*sin(u[1])-sin(u[3])*cos(u[1])
  22 : Fcn  Expr=sin(u[3])*sin(u[2])*sin(u[1])+cos(u[3])*cos(u[1])
  23 : Fcn  Expr=cos(u[2])*sin(u[1])
  31 : Fcn  Expr=cos(u[3])*sin(u[2])*cos(u[1])+sin(u[3])*sin(u[1])
  32 : Fcn  Expr=sin(u[3])*sin(u[2])*cos(u[1])-cos(u[3])*sin(u[1])
  33 : Fcn  Expr=cos(u[2])*cos(u[1])
  Mux2 : Mux  Inputs=9
  Reshape : Reshape  OutputDimensionality=Customize  OutputDimensions=[3,3]
  Rot : Outport
  wires:
  33/1 -> Mux2/9
  32/1 -> Mux2/8
  31/1 -> Mux2/7
  23/1 -> Mux2/6
  22/1 -> Mux2/5
  21/1 -> Mux2/4
  13/1 -> Mux2/3
  12/1 -> Mux2/2
  11/1 -> Mux2/1
  Mux2/1 -> Reshape/1
  Euler/1 -> 11/1, 33/1, 32/1, 31/1, 23/1, 22/1, 21/1, 13/1, 12/1
  Reshape/1 -> Rot/1

== system InnerOuter_Sim_newNav/6DOF Model/Plant/6-DOF EOM/[V1,2,3,W1,2,3] ==
  note: V*dot =Inv(A){[F ; M] - SigmaAV*}
  "[F ; M]" : Inport
  Euler : Inport  Port=2
  V* : Inport  Port=3  PortDimensions=6
  A = [M ; J] : Subsystem
  Acc_meas : Product  Inputs=/*  Multiplication=Matrix(*)  SaturateOnIntegerOverflow=on  InputSameDT=on  OutDataTypeStr=Inherit: Same as first input
  Demux : Demux  Outputs=[3;3]
  Get Grav Force in Body : Subsystem
  Gravitational Acc : Constant  Value=[0 0 -ISA_g]  VectorParams1D=off
  Selector3 : Selector  InputPortWidth=6  IndexOptions=Index vector (dialog)  Indices=1:3  OutputSizes=1
  Sigma : Subsystem
  Sigma*A : Product  Multiplication=Matrix(*)  SaturateOnIntegerOverflow=on  InputSameDT=on  OutDataTypeStr=Inherit: Same as first input
  Sigma*A*V* : Product  Multiplication=Matrix(*)  SaturateOnIntegerOverflow=on  InputSameDT=on  OutDataTypeStr=Inherit: Same as first input
  Sum1 : Sum  Inputs=+-|  SaturateOnIntegerOverflow=on  InputSameDT=on  OutDataTypeStr=Inherit: Same as first input
  Sum2 : Sum  Inputs=++|  SaturateOnIntegerOverflow=on  InputSameDT=on  OutDataTypeStr=Inherit: Same as first input
  Terminator1 : Terminator
  "V*dot " : Product  Inputs=/*  Multiplication=Matrix(*)  SaturateOnIntegerOverflow=on  InputSameDT=on  OutDataTypeStr=Inherit: Same as first input
  "Acc_meas " : Outport
  V*dot : Outport  Port=2
  wires:
  Sum2/1 -> "Acc_meas "/1
  Get Grav Force in Body/1(Grav Force (Body)) -> Sum2/1
  Selector3/1 -> Sum2/2
  Euler/1 -> Get Grav Force in Body/1(Euler)
  Gravitational Acc/1 -> Get Grav Force in Body/2(Grav Force)
  Acc_meas/1 -> Selector3/1
  Sigma*A/1 -> Sigma*A*V*/1
  "V*dot "/1 -> V*dot/1
  V*/1 -> Demux/1, Sigma*A*V*/2
  Demux/2 -> Sigma/1(pqr)
  Sigma*A*V*/1 -> Sum1/2
  "[F ; M]"/1 -> Acc_meas/2, Sum1/1
  Sigma/1(Sigma) -> Sigma*A/1
  Demux/1 -> Terminator1/1
  A = [M ; J]/1(A Matrix) -> Acc_meas/1, "V*dot "/1, Sigma*A/2
  Sum1/1 -> "V*dot "/2

== system InnerOuter_Sim_newNav/6DOF Model/Plant/Engine Model/Get To1 ==
  dt : Inport
  Divide : Product  Inputs=3
  Math Function : Math  Operator=pow  SaturateOnIntegerOverflow=on
  Math Function1 : Math  Operator=pow  SaturateOnIntegerOverflow=on
  MaxRPM : Gain  Gain=7200  SaturateOnIntegerOverflow=on  OutDataTypeStr=Inherit: Same as input  ParamDataTypeStr=Inherit: Same as input
  Min RPM : Constant  Value=2000
  Min Th K : Constant  Value=MinThK
  Prop Diameter (in) : Constant  Value=17
  Prop Diameter (in)1 : Constant  Value=2
  Prop Diameter (in)2 : Constant  Value=4
  Saturation : Saturate  UpperLimit=1.0  LowerLimit=0
  Sum : Sum  Inputs=|++
  Sum1 : Sum  Inputs=|++
  TFact : simulink/Math Operations/Slider Gain  low=0  gain=0.2  high=1
  Th K : Gain  Gain=ThK  SaturateOnIntegerOverflow=on  OutDataTypeStr=Inherit: Same as input  ParamDataTypeStr=Inherit: Same as input
  To Constant : Constant  Value=2.83e-12
  To : Outport
  wires:
  Saturation/1 -> Th K/1
  Prop Diameter (in)1/1 -> Math Function/2
  Prop Diameter (in)2/1 -> Math Function1/2
  Prop Diameter (in)/1 -> Math Function1/1
  Math Function/1 -> Divide/1
  Math Function1/1 -> Divide/2
  To Constant/1 -> Divide/3
  Divide/1 -> TFact/1
  TFact/1 -> To/1
  Sum/1 -> Math Function/1
  Min RPM/1 -> Sum/2
  MaxRPM/1 -> Sum/1
  Th K/1 -> Sum1/1
  dt/1 -> Saturation/1
  Sum1/1 -> MaxRPM/1
  Min Th K/1 -> Sum1/2

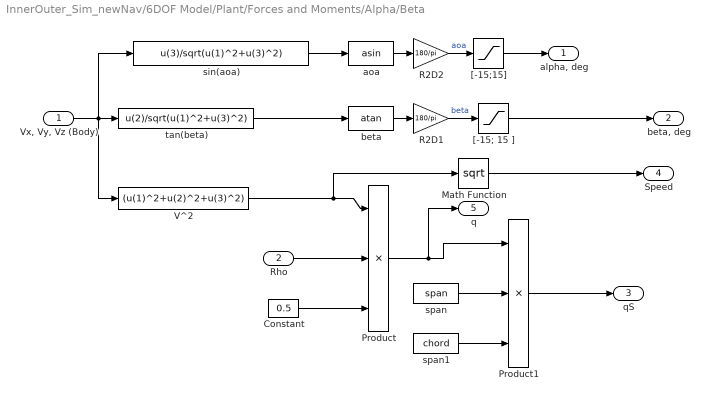
== system InnerOuter_Sim_newNav/6DOF Model/Plant/Forces and Moments/Alpha/Beta ==
  "Vx, Vy, Vz (Body)" : Inport
  Rho : Inport  Port=2
  Constant : Constant  Value=0.5  VectorParams1D=off
  Math Function : Math  Operator=sqrt  SaturateOnIntegerOverflow=on
  Product : Product  Inputs=3  SaturateOnIntegerOverflow=on  OutDataTypeStr=Inherit: Same as first input
  Product1 : Product  Inputs=3  SaturateOnIntegerOverflow=on  OutDataTypeStr=Inherit: Same as first input
  R2D1 : Gain  Gain=180/pi  SaturateOnIntegerOverflow=on  OutDataTypeStr=Inherit: Same as input  ParamDataTypeStr=Inherit: Same as input
  R2D2 : Gain  Gain=180/pi  SaturateOnIntegerOverflow=on  OutDataTypeStr=Inherit: Same as input  ParamDataTypeStr=Inherit: Same as input
  V^2 : Fcn  Expr=(u(1)^2+u(2)^2+u(3)^2)
  "[-15; 15 ]" : Saturate  UpperLimit=15  LowerLimit=-15
  "[-15;15]" : Saturate  UpperLimit=15  LowerLimit=-15
  aoa : Trigonometry  Operator=asin
  beta : Trigonometry  Operator=atan
  sin(aoa) : Fcn  Expr=u(3)/sqrt(u(1)^2+u(3)^2)
  span : Constant  Value=span  VectorParams1D=off
  span1 : Constant  Value=chord  VectorParams1D=off
  tan(beta) : Fcn  Expr=u(2)/sqrt(u(1)^2+u(3)^2)
  "alpha, deg" : Outport
  "beta, deg" : Outport  Port=2
  qS : Outport  Port=3
  Speed : Outport  Port=4
  q : Outport  Port=5
  wires:
  Product/1 -> q/1, Product1/1
  Product1/1 -> qS/1
  span1/1 -> Product1/3
  span/1 -> Product1/2
  "Vx, Vy, Vz (Body)"/1 -> sin(aoa)/1, V^2/1, tan(beta)/1
  tan(beta)/1 -> beta/1
  beta/1 -> R2D1/1
  V^2/1 -> Product/1, Math Function/1
  Rho/1 -> Product/2
  Constant/1 -> Product/3
  R2D1/1 -> "[-15; 15 ]"/1  "beta"
  aoa/1 -> R2D2/1
  R2D2/1 -> "[-15;15]"/1  "aoa"
  sin(aoa)/1 -> aoa/1
  Math Function/1 -> Speed/1
  "[-15;15]"/1 -> "alpha, deg"/1
  "[-15; 15 ]"/1 -> "beta, deg"/1

== system InnerOuter_Sim_newNav/6DOF Model/Plant/Forces and Moments/Body Frame F & M ==
  "Alpha, deg" : Inport
  "Beta, deg" : Inport  Port=2
  qs : Inport  Port=3
  Airspeed : Inport  Port=4
  "de, deg" : Inport  Port=5
  "daL, deg" : Inport  Port=6
  "daR, deg" : Inport  Port=7
  "dr, deg" : Inport  Port=8
  "df, deg" : Inport  Port=9
  p,q,r : Inport  Port=10
  Bus Creator : BusCreator  Inputs=2
  Transfer to body frame : Subsystem
  Wind frame F& M : Subsystem
  F_b : Outport
  M_b : Outport  Port=2
  wires:
  "Alpha, deg"/1 -> Wind frame F& M/1("alpha, deg"), Bus Creator/1
  "Beta, deg"/1 -> Wind frame F& M/2("beta, deg"), Bus Creator/2
  "dr, deg"/1 -> Wind frame F& M/6("dr, deg")
  "daL, deg"/1 -> Wind frame F& M/4("daL, deg")
  "de, deg"/1 -> Wind frame F& M/3("de, deg")
  Wind frame F& M/1(F&M wind frame) -> Transfer to body frame/1(Wind frame  F&M)
  Bus Creator/1 -> Transfer to body frame/2("aoa/beta, deg")  "aoa/beta, deg"
  Transfer to body frame/1(F_b) -> F_b/1
  Transfer to body frame/2(M_b) -> M_b/1
  "df, deg"/1 -> Wind frame F& M/7("df, deg")
  qs/1 -> Wind frame F& M/8(qS)
  p,q,r/1 -> Wind frame F& M/9(p,q,r)
  Airspeed/1 -> Wind frame F& M/10(Airpseed)
  "daR, deg"/1 -> Wind frame F& M/5("daR, deg")

== system InnerOuter_Sim_newNav/6DOF Model/Plant/Forces and Moments/Get Grav Force in Body ==
  Euler : Inport
  Grav Force : Inport  Port=2
  Math Function : Math  Operator=transpose  SaturateOnIntegerOverflow=on
  Product1 : Product  Multiplication=Matrix(*)  SaturateOnIntegerOverflow=on  InputSameDT=on  OutDataTypeStr=Inherit: Same as first input
  Rb2u : Subsystem
  Reshape : Reshape  OutputDimensionality=Column vector (2-D)
  Grav Force (Body) : Outport
  wires:
  Rb2u/1(DCM) -> Math Function/1
  Euler/1 -> Rb2u/1(phi theta psi)
  Product1/1 -> Grav Force (Body)/1
  Math Function/1 -> Product1/1
  Grav Force/1 -> Reshape/1
  Reshape/1 -> Product1/2

== system InnerOuter_Sim_newNav/6DOF Model/Plant/Forces and Moments/NED(u)2b ==
  V w : Inport
  Euler : Inport  Port=2
  RB2LTP : Subsystem
  RL2B * Vw : Product  Multiplication=Matrix(*)  SaturateOnIntegerOverflow=on  InputSameDT=on  OutDataTypeStr=Inherit: Same as first input
  RLTP2B : Math  Operator=transpose  SaturateOnIntegerOverflow=on
  Reshape1 : Reshape  OutputDimensionality=Row vector (2-D)
  Vb Corr : Outport
  wires:
  RL2B * Vw/1 -> Reshape1/1
  Euler/1 -> RB2LTP/1(Euler)
  RB2LTP/1(RB2L) -> RLTP2B/1
  RLTP2B/1 -> RL2B * Vw/1
  V w/1 -> RL2B * Vw/2
  Reshape1/1 -> Vb Corr/1

== system InnerOuter_Sim_newNav/6DOF Model/Plant/Magnetometer/RB2LTP ==
  Euler : Inport
  11 : Fcn  Expr=cos(u[3])*cos(u[2])
  12 : Fcn  Expr=sin(u[3])*cos(u[2])
  13 : Fcn  Expr=-sin(u[2])
  21 : Fcn  Expr=cos(u[3])*sin(u[2])*sin(u[1])-sin(u[3])*cos(u[1])
  22 : Fcn  Expr=sin(u[3])*sin(u[2])*sin(u[1])+cos(u[3])*cos(u[1])
  23 : Fcn  Expr=cos(u[2])*sin(u[1])
  31 : Fcn  Expr=cos(u[3])*sin(u[2])*cos(u[1])+sin(u[3])*sin(u[1])
  32 : Fcn  Expr=sin(u[3])*sin(u[2])*cos(u[1])-cos(u[3])*sin(u[1])
  33 : Fcn  Expr=cos(u[2])*cos(u[1])
  Mux2 : Mux  Inputs=9
  Reshape : Reshape  OutputDimensionality=Customize  OutputDimensions=[3,3]
  Rot : Outport
  wires:
  33/1 -> Mux2/9
  32/1 -> Mux2/8
  31/1 -> Mux2/7
  23/1 -> Mux2/6
  22/1 -> Mux2/5
  21/1 -> Mux2/4
  13/1 -> Mux2/3
  12/1 -> Mux2/2
  11/1 -> Mux2/1
  Mux2/1 -> Reshape/1
  Euler/1 -> 11/1, 33/1, 32/1, 31/1, 23/1, 22/1, 21/1, 13/1, 12/1
  Reshape/1 -> Rot/1

== system InnerOuter_Sim_newNav/6DOF Model/Plant/[0, pi] Wrap Around/Negative Yaw ==
  yaw : Inport
  Enable : EnablePort
  Abs : Abs
  Constant1 : Constant  Value=2*pi
  Constant2 : Constant  Value=2*pi
  Math Function : Math  Operator=mod  SaturateOnIntegerOverflow=on
  Sum : Sum  Inputs=|-+
  yaw_wr : Outport
  wires:
  yaw/1 -> Abs/1
  Constant1/1 -> Math Function/2
  Math Function/1 -> Sum/1
  Abs/1 -> Math Function/1
  Constant2/1 -> Sum/2
  Sum/1 -> yaw_wr/1

== system InnerOuter_Sim_newNav/6DOF Model/Plant/[0, pi] Wrap Around/Positive Yaw ==
  yaw : Inport
  Enable : EnablePort
  Constant1 : Constant  Value=2*pi
  Math Function : Math  Operator=mod  SaturateOnIntegerOverflow=on
  yaw_wr : Outport
  wires:
  yaw/1 -> Math Function/1
  Constant1/1 -> Math Function/2
  Math Function/1 -> yaw_wr/1

== system InnerOuter_Sim_newNav/L1 Output Feedback Controller With  Projection Operator/Control  Law/Compute Coef/Subsystem11 ==
  u : Inport
  Environment Controller : simulink/Signal Routing/Environment Controller
  Math Function : Math  SaturateOnIntegerOverflow=on
  exp(u) : Outport
  wires:
  Environment Controller/1 -> exp(u)/1
  Math Function/1 -> Environment Controller/1
  u/1 -> Math Function/1

== system InnerOuter_Sim_newNav/L1 Output Feedback Controller With  Projection Operator/State Predictor/Compute Coef/Subsystem11 ==
  u : Inport
  Environment Controller : simulink/Signal Routing/Environment Controller
  Math Function : Math  SaturateOnIntegerOverflow=on
  exp(u) : Outport
  wires:
  Environment Controller/1 -> exp(u)/1
  Math Function/1 -> Environment Controller/1
  u/1 -> Math Function/1

== system InnerOuter_Sim_newNav/6DOF Model/Plant/6-DOF EOM/[V1,2,3,W1,2,3]/A = [M ; J] ==
  Constant1 : Constant  Value=zeros(3,3)
  Constant4 : Constant  Value=0
  Display : Display
  Display1 : Display
  Display2 : Display
  Ixx : Constant  Value=Ixx  VectorParams1D=off
  Iyy : Constant  Value=Iyy  VectorParams1D=off
  Izz : Constant  Value=Izz  VectorParams1D=off
  Matrix Concatenation : Concatenate  Mode=Multidimensional array
  Matrix Concatenation1 : Concatenate  Mode=Multidimensional array
  Matrix Concatenation2 : Concatenate  Mode=Multidimensional array  ConcatenateDimension=2
  Mux : Mux  Inputs=9
  Mux1 : Mux  Inputs=9
  Reshape : Reshape  OutputDimensionality=Customize  OutputDimensions=[3,3]
  Reshape1 : Reshape  OutputDimensionality=Customize  OutputDimensions=[3,3]
  mass : Constant  Value=mass  VectorParams1D=off
  A Matrix : Outport
  wires:
  Ixx/1 -> Mux/1
  Izz/1 -> Mux/9
  Iyy/1 -> Mux/5
  Constant4/1 -> Mux/8, Mux/7, Mux/6, Mux/4, Mux/3, Mux/2, Mux1/8, Mux1/7, Mux1/6, Mux1/4, Mux1/3, Mux1/2
  mass/1 -> Mux1/1, Mux1/5, Mux1/9
  Mux1/1 -> Reshape/1
  Mux/1 -> Reshape1/1
  Matrix Concatenation/1 -> Matrix Concatenation2/1, Display/1
  Matrix Concatenation1/1 -> Matrix Concatenation2/2, Display1/1
  Matrix Concatenation2/1 -> A Matrix/1, Display2/1
  Reshape1/1 -> Matrix Concatenation1/2
  Reshape/1 -> Matrix Concatenation/1
  Constant1/1 -> Matrix Concatenation/2, Matrix Concatenation1/1

== system InnerOuter_Sim_newNav/6DOF Model/Plant/6-DOF EOM/[V1,2,3,W1,2,3]/Get Grav Force in Body ==
  Euler : Inport
  Grav Force : Inport  Port=2
  Math Function : Math  Operator=transpose  SaturateOnIntegerOverflow=on
  Product1 : Product  Multiplication=Matrix(*)  SaturateOnIntegerOverflow=on  InputSameDT=on  OutDataTypeStr=Inherit: Same as first input
  Rb2u : Subsystem
  Reshape : Reshape  OutputDimensionality=Column vector (2-D)
  Grav Force (Body) : Outport
  wires:
  Rb2u/1(DCM) -> Math Function/1
  Euler/1 -> Rb2u/1(phi theta psi)
  Product1/1 -> Grav Force (Body)/1
  Math Function/1 -> Product1/1
  Grav Force/1 -> Reshape/1
  Reshape/1 -> Product1/2
